simulink model "CommanderBlock"  (R2020b)
settings: Solver=VariableStepAuto  StartTime=0.0  StopTime=10.0  RelTol=1e-3
undefined symbols (not defined in the file or in its folder): cam_control_gain, l_stick_x_gain, l_stick_y_gain, m, r_stick_x_gain, r_stick_y_gain, x_final, y_final, z_final
libraries: pid_lib x4, aerolibguid x1
settings Model: Creator=macra  LastModifiedBy=macra

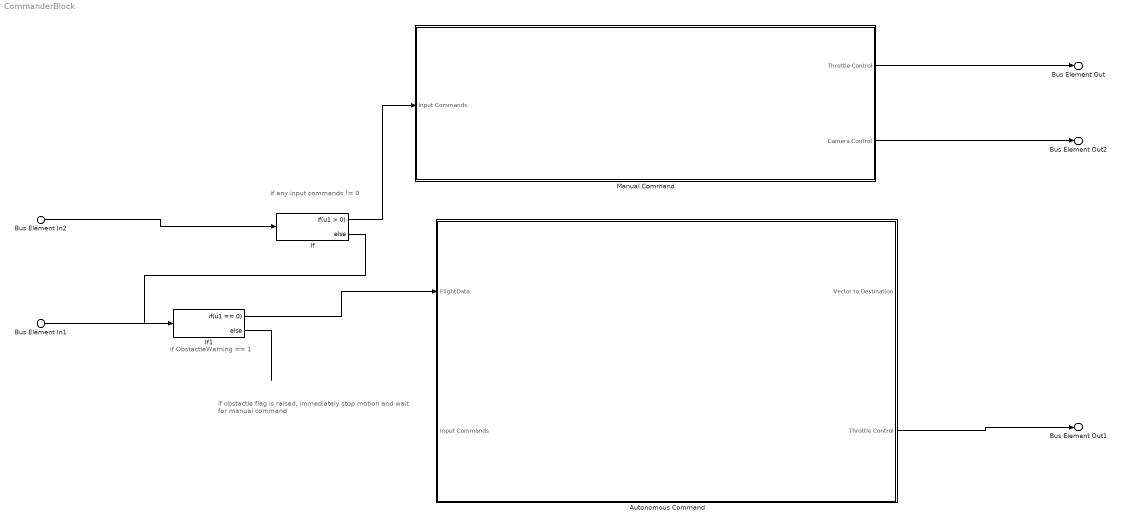
== system CommanderBlock ==
  note: if ObstactleWarning == 1
  note: if any input commands != 0
  note: if obstactle flag is raised,
      | immediately stop motion and wait for manual command
  Bus Element In2 : Inport  PortName=Input Commands
  Bus Element In1 : Inport  Port=2  PortName=Flight Data
  Autonomous Command : Subsystem
  If : If
  If1 : If  IfExpression=u1 == 0
  Manual Command : Subsystem
  Bus Element Out : Outport  PortName=Throttle Control  Element=signal1
  Bus Element Out1 : Outport  PortName=Throttle Control  Element=signal2
  Bus Element Out2 : Outport  Port=2  PortName=Camera Control  Element=signal1
  wires:
  Bus Element In2/1 -> If/1
  If/1 -> Manual Command/1(Input Commands)
  If1/1 -> Autonomous Command/1(FlightData)
  If1/2 -> ?
  Bus Element In1/1 -> If1/1
  Manual Command/1(Throttle Control) -> Bus Element Out/1
  Autonomous Command/2(Throttle Control) -> Bus Element Out1/1
  Manual Command/2(Camera Control) -> Bus Element Out2/1
  If/2 -> ?

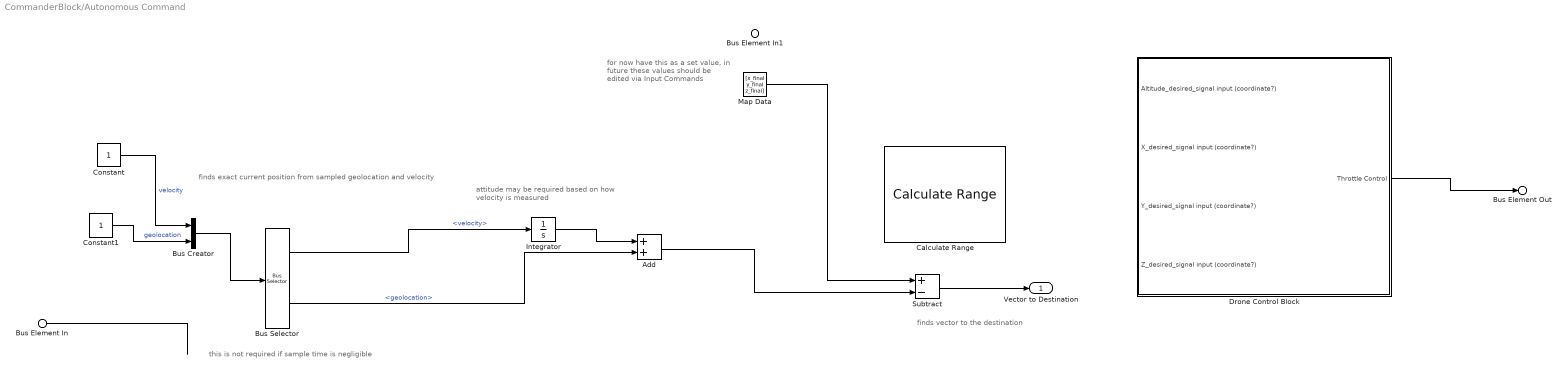
== system CommanderBlock/Autonomous Command ==
  note: finds vector to the destination
  note: finds exact current position from sampled geolocation and velocity
  note: this is not required if sample time is negligible
  note: attitude may be required based on how
      | velocity is measured
  note: for now have this as a set value,
      | in future these values should be
      | edited via Input Commands
  Bus Element In : Inport  PortName=FlightData
  Bus Element In1 : Inport  Port=2  PortName=Input Commands
  Add : Sum
  Bus Creator : BusCreator  Inputs=2
  Bus Selector : BusSelector  OutputSignals=velocity,geolocation
  Calculate Range : aerolibguid/Calculate Range
      settings: SourceProductBaseCode=AE
  Constant : Constant
  Constant1 : Constant
  Drone Control Block : Subsystem
  Integrator : Integrator
  Map Data : Constant  Value=[x_final y_final z_final]
  Subtract : Sum  Inputs=+-
  Vector to Destination : Outport
  Bus Element Out : Outport  Port=2  PortName=Throttle Control  Element=signal1
  wires:
  Constant/1 -> Bus Creator/1  "velocity"
  Bus Creator/1 -> Bus Selector/1
  Bus Selector/1 -> Integrator/1  "<velocity>"
  Constant1/1 -> Bus Creator/2  "geolocation"
  Bus Selector/2 -> Add/2  "<geolocation>"
  Integrator/1 -> Add/1
  Bus Element In/1 -> ?
  Subtract/1 -> Vector to Destination/1
  Add/1 -> Subtract/2
  Drone Control Block/1(Throttle Control) -> Bus Element Out/1
  Map Data/1 -> Subtract/1

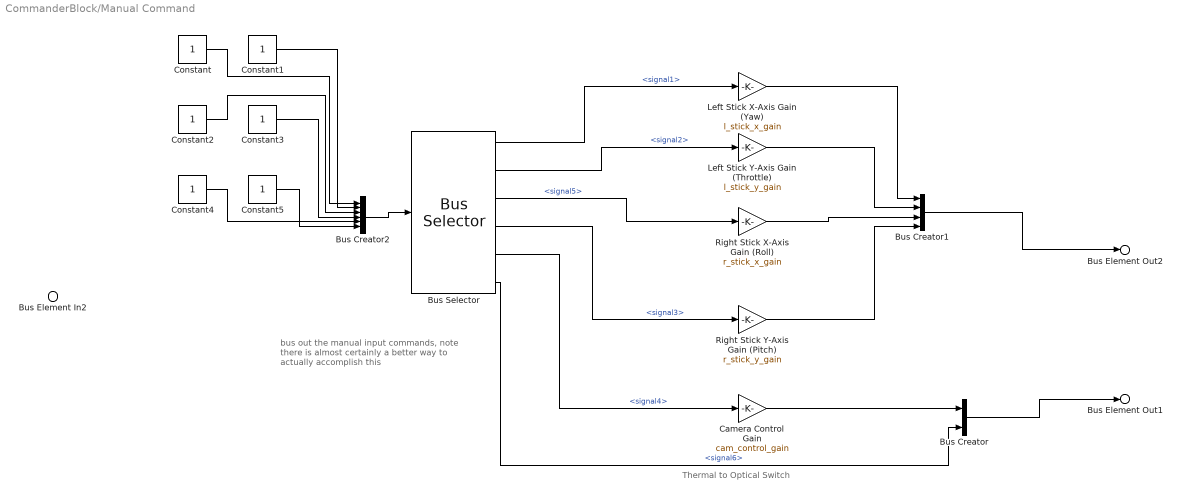
== system CommanderBlock/Manual Command ==
  note: Thermal to Optical Switch
  note: bus out the manual input commands,
      | note there is almost certainly a better way
      | to actually accomplish this
  Bus Element In2 : Inport  PortName=Input Commands
  Bus Creator : BusCreator  Inputs=2
  Bus Creator1 : BusCreator  Inputs=4
  Bus Creator2 : BusCreator  Inputs=6
  Bus Selector : BusSelector  OutputSignals=signal1,signal2,signal5,signal3,signal4,signal6
  Camera Control Gain : Gain  Gain=cam_control_gain
  Constant{,1..5} (6 alike) : Constant
  Left Stick X-Axis Gain (Yaw) : Gain  Gain=l_stick_x_gain
  Left Stick Y-Axis Gain (Throttle) : Gain  Gain=l_stick_y_gain
  Right Stick X-Axis Gain (Roll) : Gain  Gain=r_stick_x_gain
  Right Stick Y-Axis Gain (Pitch) : Gain  Gain=r_stick_y_gain
  Bus Element Out2 : Outport  PortName=Throttle Control
  Bus Element Out1 : Outport  Port=2  PortName=Camera Control
  wires:
  Constant4/1 -> Bus Creator2/5
  Constant5/1 -> Bus Creator2/6
  Bus Creator1/1 -> Bus Element Out2/1
  Bus Selector/6 -> Bus Creator/2  "<signal6>"
  Constant/1 -> Bus Creator2/1
  Constant3/1 -> Bus Creator2/4
  Right Stick Y-Axis Gain (Pitch)/1 -> Bus Creator1/4
  Bus Selector/3 -> Right Stick X-Axis Gain (Roll)/1  "<signal5>"
  Left Stick Y-Axis Gain (Throttle)/1 -> Bus Creator1/2
  Bus Selector/4 -> Right Stick Y-Axis Gain (Pitch)/1  "<signal3>"
  Bus Selector/1 -> Left Stick X-Axis Gain (Yaw)/1  "<signal1>"
  Constant1/1 -> Bus Creator2/2
  Bus Creator2/1 -> Bus Selector/1
  Bus Selector/5 -> Camera Control Gain/1  "<signal4>"
  Bus Creator/1 -> Bus Element Out1/1
  Left Stick X-Axis Gain (Yaw)/1 -> Bus Creator1/1
  Right Stick X-Axis Gain (Roll)/1 -> Bus Creator1/3
  Constant2/1 -> Bus Creator2/3
  Bus Selector/2 -> Left Stick Y-Axis Gain (Throttle)/1  "<signal2>"
  Camera Control Gain/1 -> Bus Creator/1

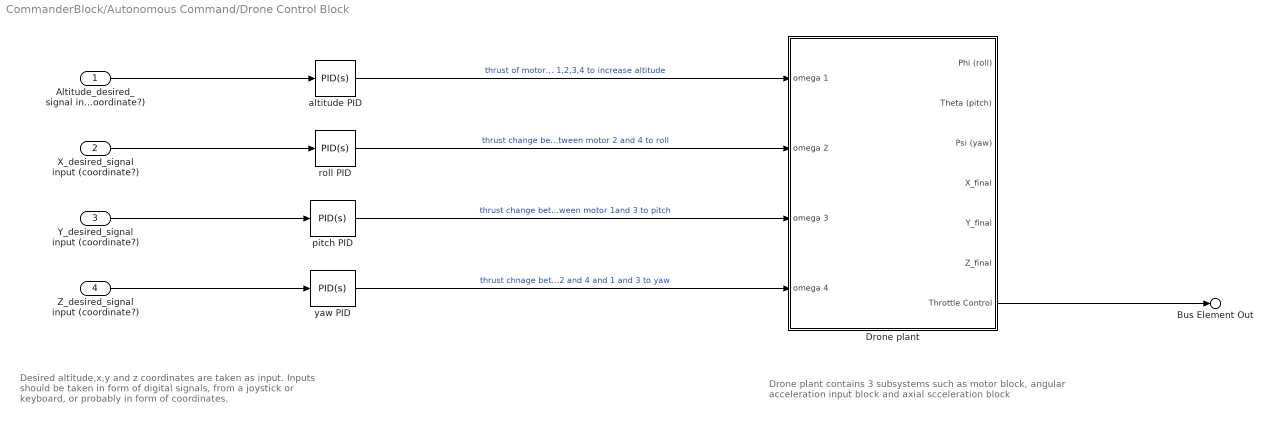
== system CommanderBlock/Autonomous Command/Drone Control Block ==
  note: Desired altitude,x,y and z coordinates are taken as input.
      | Inputs should be taken in form of digital signals,
      | from a joystick or keyboard, or probably in form of coordinates.
  note: Drone plant contains 3 subsystems such as motor block,
      | angular acceleration input block and axial scceleration block
  Altitude_desired_signal input (coordinate?) : Inport
  X_desired_signal input (coordinate?) : Inport  Port=2
  Y_desired_signal input (coordinate?) : Inport  Port=3
  Z_desired_signal input (coordinate?) : Inport  Port=4
  Drone plant : Subsystem
  altitude PID : pid_lib/PID Controller  Controller=PID  Form=Parallel  TimeDomain=Continuous-time  UseExternalTs=off  SampleTime=-1  IntegratorMethod=Forward Euler  FilterMethod=Forward Euler  ControllerParametersSource=internal  P=1  I=1  D=0  UseFilter=on  N=100  TunerSelectOption=Transfer Function Based (PID Tuner App)  InitialConditionSource=internal  InitialConditionForIntegrator=0  InitialConditionForFilter=0  DifferentiatorICPrevScaledInput=0  ExternalReset=none  TrackingMode=off  Kt=1  LimitOutput=off  SatLimitsSource=internal  UpperSaturationLimit=inf  LowerSaturationLimit=-inf  LinearizeAsGain=on  AntiWindupMode=none  Kb=1  POutMin=[]  POutMax=[]  IOutMin=[]  IOutMax=[]  DOutMin=[]  DOutMax=[]  NOutMin=[]  NOutMax=[]  SumOutMin=[]  SumOutMax=[]  SaturationOutMin=[]  SaturationOutMax=[]  PParamMin=[]  PParamMax=[]  IParamMin=[]  IParamMax=[]  DParamMin=[]  DParamMax=[]  NParamMin=[]  NParamMax=[]  KbParamMin=[]  KbParamMax=[]  KtParamMin=[]  KtParamMax=[]  KbOutMin=[]  KbOutMax=[]  KtOutMin=[]  KtOutMax=[]  IntegratorOutMin=[]  IntegratorOutMax=[]  FilterOutMin=[]  FilterOutMax=[]  SumI1OutMin=[]  SumI1OutMax=[]  SumI2OutMin=[]  SumI2OutMax=[]  SumI3OutMin=[]  SumI3OutMax=[]  SumI4OutMin=[]  SumI4OutMax=[]  SumDOutMin=[]  SumDOutMax=[]  DifferentiatorOutMin=[]  DifferentiatorOutMax=[]  FilterDiffOutCoefMin=[]  FilterDiffOutCoefMax=[]  ReciprocalOutMin=[]  ReciprocalOutMax=[]  SumDenOutMin=[]  SumDenOutMax=[]  SumNumOutMin=[]  SumNumOutMax=[]  DivideOutMin=[]  DivideOutMax=[]  UdiffTsProdOutMin=[]  UdiffTsProdOutMax=[]  NTsProdOutMin=[]  NTsProdOutMax=[]  UintegralTsProdOutMin=[]  UintegralTsProdOutMax=[]  UngainTsProdOutMin=[]  UngainTsProdOutMax=[]  IntegratorContinuousStateAttributes=''  IntegratorStateMustResolveToSignalObject=off  IntegratorRTWStateStorageClass=Auto  FilterContinuousStateAttributes=''  FilterStateMustResolveToSignalObject=off  FilterRTWStateStorageClass=Auto  ParallelPVariant=InternalParameters  IdealPVariant=Disabled  IVariant=InternalParameters  DVariant=InternalParameters  IntegratorVariant=Continuous  SatVariant=Disabled  AWVariant=Passthrough  PCopyVariant=Disabled  TRVariant=Disabled  FdbkBlocksVariant=Forward  IdealPFdbkVariant=Disabled  SatFdbkVariant=Disabled  DerivativeFilterVariant=ContFilter  NVariant=InternalParameters  NCopyVariant=Disabled  FilterICVariant=InternalICsFilter  IntegratorICVariant=InternalICs  ExternalResetVariant=Disabled  TRSumVariant=Passthrough  SumFdbkVariant=Disabled  SumVariant=Sum_PID  TsampFilterVariant=InternalTs  TsampNgainVariant=Passthrough  TsampIntegralVariant=Passthrough  ExternalSaturationOutDataTypeStr=Inherit: Same as second input
  pitch PID : pid_lib/PID Controller  Controller=PID  Form=Parallel  TimeDomain=Continuous-time  UseExternalTs=off  SampleTime=-1  IntegratorMethod=Forward Euler  FilterMethod=Forward Euler  ControllerParametersSource=internal  P=1  I=1  D=0  UseFilter=on  N=100  TunerSelectOption=Transfer Function Based (PID Tuner App)  InitialConditionSource=internal  InitialConditionForIntegrator=0  InitialConditionForFilter=0  DifferentiatorICPrevScaledInput=0  ExternalReset=none  TrackingMode=off  Kt=1  LimitOutput=off  SatLimitsSource=internal  UpperSaturationLimit=inf  LowerSaturationLimit=-inf  LinearizeAsGain=on  AntiWindupMode=none  Kb=1  POutMin=[]  POutMax=[]  IOutMin=[]  IOutMax=[]  DOutMin=[]  DOutMax=[]  NOutMin=[]  NOutMax=[]  SumOutMin=[]  SumOutMax=[]  SaturationOutMin=[]  SaturationOutMax=[]  PParamMin=[]  PParamMax=[]  IParamMin=[]  IParamMax=[]  DParamMin=[]  DParamMax=[]  NParamMin=[]  NParamMax=[]  KbParamMin=[]  KbParamMax=[]  KtParamMin=[]  KtParamMax=[]  KbOutMin=[]  KbOutMax=[]  KtOutMin=[]  KtOutMax=[]  IntegratorOutMin=[]  IntegratorOutMax=[]  FilterOutMin=[]  FilterOutMax=[]  SumI1OutMin=[]  SumI1OutMax=[]  SumI2OutMin=[]  SumI2OutMax=[]  SumI3OutMin=[]  SumI3OutMax=[]  SumI4OutMin=[]  SumI4OutMax=[]  SumDOutMin=[]  SumDOutMax=[]  DifferentiatorOutMin=[]  DifferentiatorOutMax=[]  FilterDiffOutCoefMin=[]  FilterDiffOutCoefMax=[]  ReciprocalOutMin=[]  ReciprocalOutMax=[]  SumDenOutMin=[]  SumDenOutMax=[]  SumNumOutMin=[]  SumNumOutMax=[]  DivideOutMin=[]  DivideOutMax=[]  UdiffTsProdOutMin=[]  UdiffTsProdOutMax=[]  NTsProdOutMin=[]  NTsProdOutMax=[]  UintegralTsProdOutMin=[]  UintegralTsProdOutMax=[]  UngainTsProdOutMin=[]  UngainTsProdOutMax=[]  IntegratorContinuousStateAttributes=''  IntegratorStateMustResolveToSignalObject=off  IntegratorRTWStateStorageClass=Auto  FilterContinuousStateAttributes=''  FilterStateMustResolveToSignalObject=off  FilterRTWStateStorageClass=Auto  ParallelPVariant=InternalParameters  IdealPVariant=Disabled  IVariant=InternalParameters  DVariant=InternalParameters  IntegratorVariant=Continuous  SatVariant=Disabled  AWVariant=Passthrough  PCopyVariant=Disabled  TRVariant=Disabled  FdbkBlocksVariant=Forward  IdealPFdbkVariant=Disabled  SatFdbkVariant=Disabled  DerivativeFilterVariant=ContFilter  NVariant=InternalParameters  NCopyVariant=Disabled  FilterICVariant=InternalICsFilter  IntegratorICVariant=InternalICs  ExternalResetVariant=Disabled  TRSumVariant=Passthrough  SumFdbkVariant=Disabled  SumVariant=Sum_PID  TsampFilterVariant=InternalTs  TsampNgainVariant=Passthrough  TsampIntegralVariant=Passthrough  ExternalSaturationOutDataTypeStr=Inherit: Same as second input
  roll PID : pid_lib/PID Controller  Controller=PID  Form=Parallel  TimeDomain=Continuous-time  UseExternalTs=off  SampleTime=-1  IntegratorMethod=Forward Euler  FilterMethod=Forward Euler  ControllerParametersSource=internal  P=1  I=1  D=0  UseFilter=on  N=100  TunerSelectOption=Transfer Function Based (PID Tuner App)  InitialConditionSource=internal  InitialConditionForIntegrator=0  InitialConditionForFilter=0  DifferentiatorICPrevScaledInput=0  ExternalReset=none  TrackingMode=off  Kt=1  LimitOutput=off  SatLimitsSource=internal  UpperSaturationLimit=inf  LowerSaturationLimit=-inf  LinearizeAsGain=on  AntiWindupMode=none  Kb=1  POutMin=[]  POutMax=[]  IOutMin=[]  IOutMax=[]  DOutMin=[]  DOutMax=[]  NOutMin=[]  NOutMax=[]  SumOutMin=[]  SumOutMax=[]  SaturationOutMin=[]  SaturationOutMax=[]  PParamMin=[]  PParamMax=[]  IParamMin=[]  IParamMax=[]  DParamMin=[]  DParamMax=[]  NParamMin=[]  NParamMax=[]  KbParamMin=[]  KbParamMax=[]  KtParamMin=[]  KtParamMax=[]  KbOutMin=[]  KbOutMax=[]  KtOutMin=[]  KtOutMax=[]  IntegratorOutMin=[]  IntegratorOutMax=[]  FilterOutMin=[]  FilterOutMax=[]  SumI1OutMin=[]  SumI1OutMax=[]  SumI2OutMin=[]  SumI2OutMax=[]  SumI3OutMin=[]  SumI3OutMax=[]  SumI4OutMin=[]  SumI4OutMax=[]  SumDOutMin=[]  SumDOutMax=[]  DifferentiatorOutMin=[]  DifferentiatorOutMax=[]  FilterDiffOutCoefMin=[]  FilterDiffOutCoefMax=[]  ReciprocalOutMin=[]  ReciprocalOutMax=[]  SumDenOutMin=[]  SumDenOutMax=[]  SumNumOutMin=[]  SumNumOutMax=[]  DivideOutMin=[]  DivideOutMax=[]  UdiffTsProdOutMin=[]  UdiffTsProdOutMax=[]  NTsProdOutMin=[]  NTsProdOutMax=[]  UintegralTsProdOutMin=[]  UintegralTsProdOutMax=[]  UngainTsProdOutMin=[]  UngainTsProdOutMax=[]  IntegratorContinuousStateAttributes=''  IntegratorStateMustResolveToSignalObject=off  IntegratorRTWStateStorageClass=Auto  FilterContinuousStateAttributes=''  FilterStateMustResolveToSignalObject=off  FilterRTWStateStorageClass=Auto  ParallelPVariant=InternalParameters  IdealPVariant=Disabled  IVariant=InternalParameters  DVariant=InternalParameters  IntegratorVariant=Continuous  SatVariant=Disabled  AWVariant=Passthrough  PCopyVariant=Disabled  TRVariant=Disabled  FdbkBlocksVariant=Forward  IdealPFdbkVariant=Disabled  SatFdbkVariant=Disabled  DerivativeFilterVariant=ContFilter  NVariant=InternalParameters  NCopyVariant=Disabled  FilterICVariant=InternalICsFilter  IntegratorICVariant=InternalICs  ExternalResetVariant=Disabled  TRSumVariant=Passthrough  SumFdbkVariant=Disabled  SumVariant=Sum_PID  TsampFilterVariant=InternalTs  TsampNgainVariant=Passthrough  TsampIntegralVariant=Passthrough  ExternalSaturationOutDataTypeStr=Inherit: Same as second input
  yaw PID : pid_lib/PID Controller  Controller=PID  Form=Parallel  TimeDomain=Continuous-time  UseExternalTs=off  SampleTime=-1  IntegratorMethod=Forward Euler  FilterMethod=Forward Euler  ControllerParametersSource=internal  P=1  I=1  D=0  UseFilter=on  N=100  TunerSelectOption=Transfer Function Based (PID Tuner App)  InitialConditionSource=internal  InitialConditionForIntegrator=0  InitialConditionForFilter=0  DifferentiatorICPrevScaledInput=0  ExternalReset=none  TrackingMode=off  Kt=1  LimitOutput=off  SatLimitsSource=internal  UpperSaturationLimit=inf  LowerSaturationLimit=-inf  LinearizeAsGain=on  AntiWindupMode=none  Kb=1  POutMin=[]  POutMax=[]  IOutMin=[]  IOutMax=[]  DOutMin=[]  DOutMax=[]  NOutMin=[]  NOutMax=[]  SumOutMin=[]  SumOutMax=[]  SaturationOutMin=[]  SaturationOutMax=[]  PParamMin=[]  PParamMax=[]  IParamMin=[]  IParamMax=[]  DParamMin=[]  DParamMax=[]  NParamMin=[]  NParamMax=[]  KbParamMin=[]  KbParamMax=[]  KtParamMin=[]  KtParamMax=[]  KbOutMin=[]  KbOutMax=[]  KtOutMin=[]  KtOutMax=[]  IntegratorOutMin=[]  IntegratorOutMax=[]  FilterOutMin=[]  FilterOutMax=[]  SumI1OutMin=[]  SumI1OutMax=[]  SumI2OutMin=[]  SumI2OutMax=[]  SumI3OutMin=[]  SumI3OutMax=[]  SumI4OutMin=[]  SumI4OutMax=[]  SumDOutMin=[]  SumDOutMax=[]  DifferentiatorOutMin=[]  DifferentiatorOutMax=[]  FilterDiffOutCoefMin=[]  FilterDiffOutCoefMax=[]  ReciprocalOutMin=[]  ReciprocalOutMax=[]  SumDenOutMin=[]  SumDenOutMax=[]  SumNumOutMin=[]  SumNumOutMax=[]  DivideOutMin=[]  DivideOutMax=[]  UdiffTsProdOutMin=[]  UdiffTsProdOutMax=[]  NTsProdOutMin=[]  NTsProdOutMax=[]  UintegralTsProdOutMin=[]  UintegralTsProdOutMax=[]  UngainTsProdOutMin=[]  UngainTsProdOutMax=[]  IntegratorContinuousStateAttributes=''  IntegratorStateMustResolveToSignalObject=off  IntegratorRTWStateStorageClass=Auto  FilterContinuousStateAttributes=''  FilterStateMustResolveToSignalObject=off  FilterRTWStateStorageClass=Auto  ParallelPVariant=InternalParameters  IdealPVariant=Disabled  IVariant=InternalParameters  DVariant=InternalParameters  IntegratorVariant=Continuous  SatVariant=Disabled  AWVariant=Passthrough  PCopyVariant=Disabled  TRVariant=Disabled  FdbkBlocksVariant=Forward  IdealPFdbkVariant=Disabled  SatFdbkVariant=Disabled  DerivativeFilterVariant=ContFilter  NVariant=InternalParameters  NCopyVariant=Disabled  FilterICVariant=InternalICsFilter  IntegratorICVariant=InternalICs  ExternalResetVariant=Disabled  TRSumVariant=Passthrough  SumFdbkVariant=Disabled  SumVariant=Sum_PID  TsampFilterVariant=InternalTs  TsampNgainVariant=Passthrough  TsampIntegralVariant=Passthrough  ExternalSaturationOutDataTypeStr=Inherit: Same as second input
  Bus Element Out : Outport  PortName=Throttle Control  Element=signal1
  wires:
  Altitude_desired_signal input (coordinate?)/1 -> altitude PID/1
  pitch PID/1 -> Drone plant/3(omega 3)  "thrust change between motor 1and 3 to pitch"
  Y_desired_signal input (coordinate?)/1 -> pitch PID/1
  yaw PID/1 -> Drone plant/4(omega 4)  "thrust chnage between motor 2 and 4 and 1 and 3 to yaw"
  Drone plant/7(Throttle Control) -> Bus Element Out/1
  Z_desired_signal input (coordinate?)/1 -> yaw PID/1
  X_desired_signal input (coordinate?)/1 -> roll PID/1
  roll PID/1 -> Drone plant/2(omega 2)  "thrust change between motor 2 and 4 to roll"
  altitude PID/1 -> Drone plant/1(omega 1)  "thrust of motor 1,2,3,4 to increase altitude"

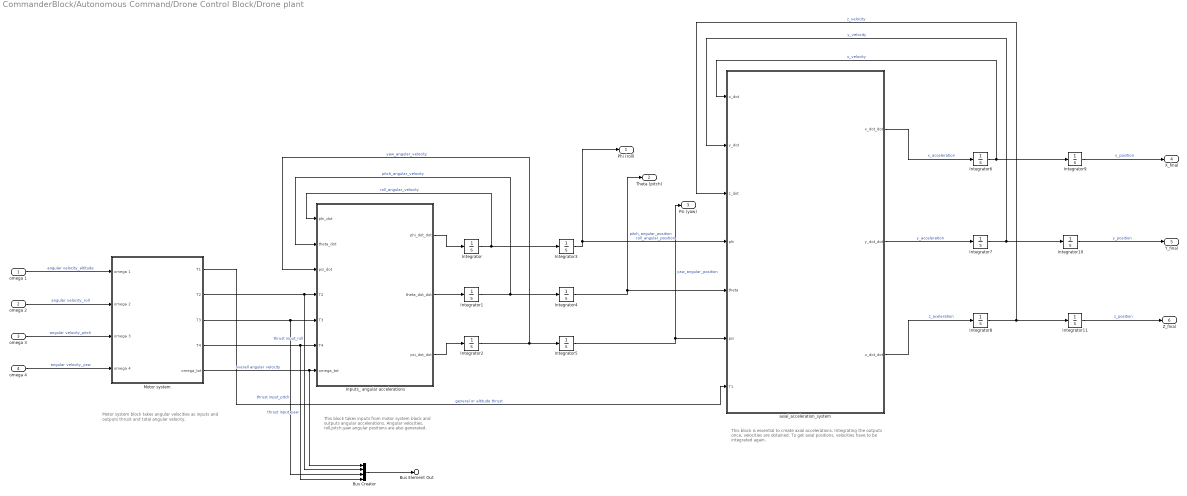
== system CommanderBlock/Autonomous Command/Drone Control Block/Drone plant ==
  note: This block is essential to create axial accelerations. Integrating the outputs
      | once, velocities are obtained. To get axial positions, velocities have to be
      | integrated again.
  note: This block takes inputs from motor system block
      | and outputs angular accelerations. Angular velocities,
      | roll,pitch,yaw angular positions are also generated.
  note: Motor system block takes angular velocities as inputs
      | and outputs thrust and total angular velocity.
  omega 1 : Inport
  omega 2 : Inport  Port=2
  omega 3 : Inport  Port=3
  omega 4 : Inport  Port=4
  Bus Creator : BusCreator  Inputs=4
  Inputs_ angular accelerations : Subsystem
  Integrator{,1..11} (12 alike) : Integrator
  Motor system : Subsystem
  axial_acceleration_system : Subsystem
  Phi (roll) : Outport
  Theta (pitch) : Outport  Port=2
  Psi (yaw) : Outport  Port=3
  X_final : Outport  Port=4
  Y_final : Outport  Port=5
  Z_final : Outport  Port=6
  Bus Element Out : Outport  Port=7  PortName=Throttle Control  Element=signal1
  wires:
  omega 1/1 -> Motor system/1(omega 1)  "angular velocity_altitude"
  omega 2/1 -> Motor system/2(omega 2)  "angular velocity_roll"
  omega 3/1 -> Motor system/3(omega 3)  "angular velocity_pitch"
  omega 4/1 -> Motor system/4(omega 4)  "angular velocity_yaw"
  Motor system/5(omega_tot) -> Bus Creator/1, Inputs_ angular accelerations/7(omega_tot)  "overall angular velocity"
  Motor system/2(T2) -> Bus Creator/2, Inputs_ angular accelerations/4(T2)  "thrust input_roll"
  Motor system/3(T3) -> Bus Creator/3, Inputs_ angular accelerations/5(T3)  "thrust input_pitch"
  Motor system/4(T4) -> Bus Creator/4, Inputs_ angular accelerations/6(T4)  "thrust input_yaw"
  Motor system/1(T1) -> axial_acceleration_system/7(T1)  "general or altitude thrust"
  Inputs_ angular accelerations/1(phi_dot_dot) -> Integrator/1
  Integrator/1 -> Inputs_ angular accelerations/1(phi_dot), Integrator3/1  "roll_angular_velocity"
  Integrator1/1 -> Inputs_ angular accelerations/2(theta_dot), Integrator4/1  "pitch_angular_velocity"
  Integrator2/1 -> Inputs_ angular accelerations/3(psi_dot), Integrator5/1  "yaw_angular_velocity"
  Inputs_ angular accelerations/2(theta_dot_dot) -> Integrator1/1
  Inputs_ angular accelerations/3(psi_dot_dot) -> Integrator2/1
  Integrator4/1 -> Theta (pitch)/1, axial_acceleration_system/5(theta)  "pitch_angular_position"
  Integrator3/1 -> Phi (roll)/1, axial_acceleration_system/4(phi)  "roll_angular_position"
  Integrator5/1 -> axial_acceleration_system/6(psi), Psi (yaw)/1  "yaw_angular_position"
  axial_acceleration_system/1(x_dot_dot) -> Integrator6/1  "x_acceleration"
  axial_acceleration_system/2(y_dot_dot) -> Integrator7/1  "y_acceleration"
  axial_acceleration_system/3(z_dot_dot) -> Integrator8/1  "z_aceleration"
  Integrator6/1 -> axial_acceleration_system/1(x_dot), Integrator9/1  "x_velocity"
  Integrator9/1 -> X_final/1  "x_position"
  Integrator7/1 -> axial_acceleration_system/2(y_dot), Integrator10/1  "y_velocity"
  Integrator10/1 -> Y_final/1  "y_position"
  Integrator8/1 -> axial_acceleration_system/3(z_dot), Integrator11/1  "z_velocity"
  Integrator11/1 -> Z_final/1  "z_position"
  Bus Creator/1 -> Bus Element Out/1

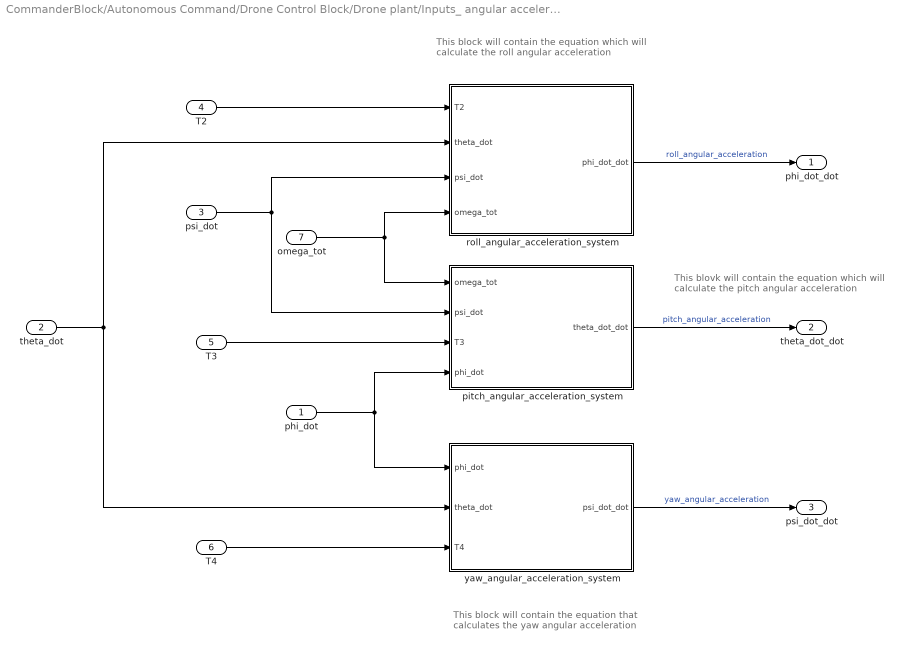
== system CommanderBlock/Autonomous Command/Drone Control Block/Drone plant/Inputs_ angular accelerations ==
  note: This blovk will contain the equation
      | which will calculate the pitch angular acceleration
  note: This block will contain the equation
      | that calculates the yaw angular acceleration
  note: This block will contain the equation
      | which will calculate the roll angular acceleration
  phi_dot : Inport
  theta_dot : Inport  Port=2
  psi_dot : Inport  Port=3
  T2 : Inport  Port=4
  T3 : Inport  Port=5
  T4 : Inport  Port=6
  omega_tot : Inport  Port=7
  pitch_angular_acceleration_system : Subsystem
  roll_angular_acceleration_system : Subsystem
  yaw_angular_acceleration_system : Subsystem
  phi_dot_dot : Outport
  theta_dot_dot : Outport  Port=2
  psi_dot_dot : Outport  Port=3
  wires:
  roll_angular_acceleration_system/1(phi_dot_dot) -> phi_dot_dot/1  "roll_angular_acceleration"
  pitch_angular_acceleration_system/1(theta_dot_dot) -> theta_dot_dot/1  "pitch_angular_acceleration"
  yaw_angular_acceleration_system/1(psi_dot_dot) -> psi_dot_dot/1  "yaw_angular_acceleration"
  T2/1 -> roll_angular_acceleration_system/1(T2)
  theta_dot/1 -> yaw_angular_acceleration_system/2(theta_dot), roll_angular_acceleration_system/2(theta_dot)
  psi_dot/1 -> roll_angular_acceleration_system/3(psi_dot), pitch_angular_acceleration_system/2(psi_dot)
  T3/1 -> pitch_angular_acceleration_system/3(T3)
  T4/1 -> yaw_angular_acceleration_system/3(T4)
  phi_dot/1 -> yaw_angular_acceleration_system/1(phi_dot), pitch_angular_acceleration_system/4(phi_dot)
  omega_tot/1 -> pitch_angular_acceleration_system/1(omega_tot), roll_angular_acceleration_system/4(omega_tot)

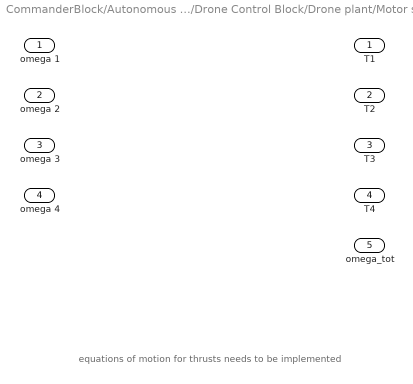
== system CommanderBlock/Autonomous Command/Drone Control Block/Drone plant/Motor system ==
  note: equations of motion for thrusts needs to be implemented
  omega 1 : Inport
  omega 2 : Inport  Port=2
  omega 3 : Inport  Port=3
  omega 4 : Inport  Port=4
  T1 : Outport
  T2 : Outport  Port=2
  T3 : Outport  Port=3
  T4 : Outport  Port=4
  omega_tot : Outport  Port=5

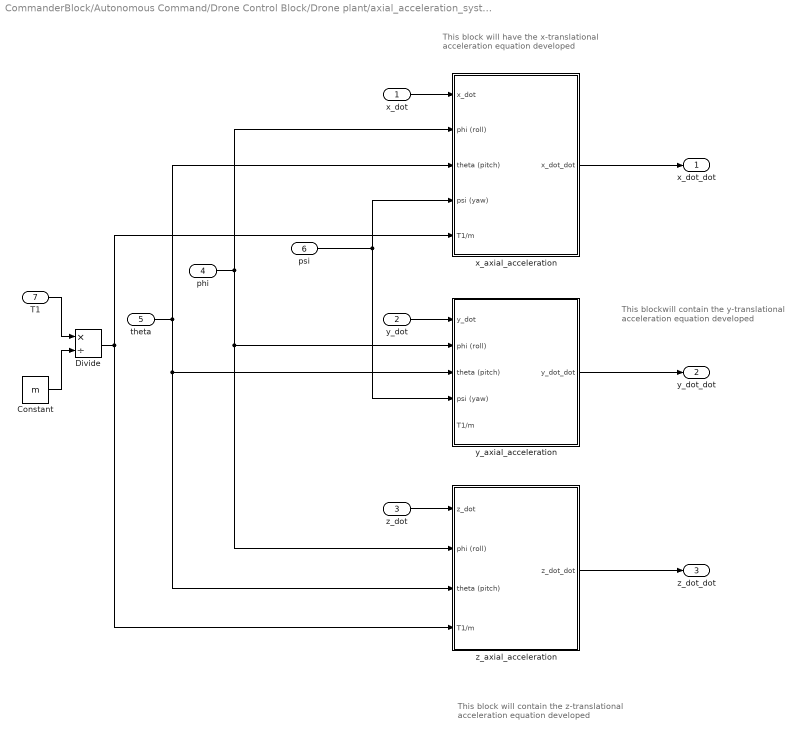
== system CommanderBlock/Autonomous Command/Drone Control Block/Drone plant/axial_acceleration_system ==
  note: This block will contain the z-translational
      | acceleration equation developed
  note: This blockwill contain the y-translational
      | acceleration equation developed
  note: This block will have the x-translational
      | acceleration equation developed
  x_dot : Inport
  y_dot : Inport  Port=2
  z_dot : Inport  Port=3
  phi : Inport  Port=4
  theta : Inport  Port=5
  psi : Inport  Port=6
  T1 : Inport  Port=7
  Constant : Constant  Value=m
  Divide : Product  Inputs=*/
  x_axial_acceleration : Subsystem
  y_axial_acceleration : Subsystem
  z_axial_acceleration : Subsystem
  x_dot_dot : Outport
  y_dot_dot : Outport  Port=2
  z_dot_dot : Outport  Port=3
  wires:
  x_axial_acceleration/1(x_dot_dot) -> x_dot_dot/1
  z_axial_acceleration/1(z_dot_dot) -> z_dot_dot/1
  y_axial_acceleration/1(y_dot_dot) -> y_dot_dot/1
  x_dot/1 -> x_axial_acceleration/1(x_dot)
  y_dot/1 -> y_axial_acceleration/1(y_dot)
  z_dot/1 -> z_axial_acceleration/1(z_dot)
  phi/1 -> y_axial_acceleration/2(phi (roll)), z_axial_acceleration/2(phi (roll)), x_axial_acceleration/2(phi (roll))
  theta/1 -> x_axial_acceleration/3(theta (pitch)), y_axial_acceleration/3(theta (pitch)), z_axial_acceleration/3(theta (pitch))
  psi/1 -> x_axial_acceleration/4(psi (yaw)), y_axial_acceleration/4(psi (yaw))
  Constant/1 -> Divide/2
  T1/1 -> Divide/1
  Divide/1 -> z_axial_acceleration/4(T1/m), x_axial_acceleration/5(T1/m)

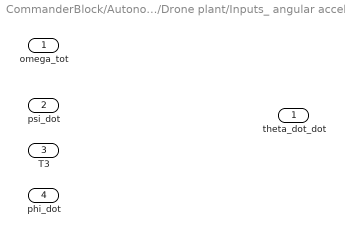
== system CommanderBlock/Autonomous Command/Drone Control Block/Drone plant/Inputs_ angular accelerations/pitch_angular_acceleration_system ==
  omega_tot : Inport
  psi_dot : Inport  Port=2
  T3 : Inport  Port=3
  phi_dot : Inport  Port=4
  theta_dot_dot : Outport

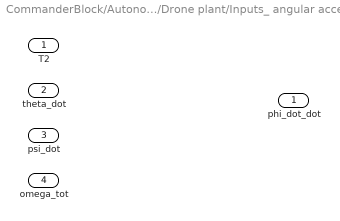
== system CommanderBlock/Autonomous Command/Drone Control Block/Drone plant/Inputs_ angular accelerations/roll_angular_acceleration_system ==
  T2 : Inport
  theta_dot : Inport  Port=2
  psi_dot : Inport  Port=3
  omega_tot : Inport  Port=4
  phi_dot_dot : Outport

== system CommanderBlock/Autonomous Command/Drone Control Block/Drone plant/Inputs_ angular accelerations/yaw_angular_acceleration_system ==
  phi_dot : Inport
  theta_dot : Inport  Port=2
  T4 : Inport  Port=3
  psi_dot_dot : Outport

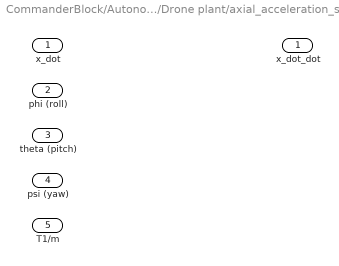
== system CommanderBlock/Autonomous Command/Drone Control Block/Drone plant/axial_acceleration_system/x_axial_acceleration ==
  x_dot : Inport
  phi (roll) : Inport  Port=2
  theta (pitch) : Inport  Port=3
  psi (yaw) : Inport  Port=4
  T1/m : Inport  Port=5
  x_dot_dot : Outport

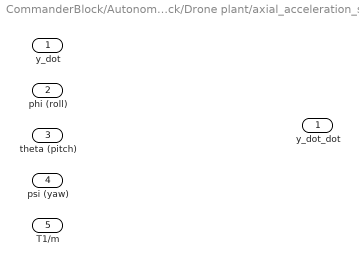
== system CommanderBlock/Autonomous Command/Drone Control Block/Drone plant/axial_acceleration_system/y_axial_acceleration ==
  y_dot : Inport
  phi (roll) : Inport  Port=2
  theta (pitch) : Inport  Port=3
  psi (yaw) : Inport  Port=4
  T1/m : Inport  Port=5
  y_dot_dot : Outport

== system CommanderBlock/Autonomous Command/Drone Control Block/Drone plant/axial_acceleration_system/z_axial_acceleration ==
  z_dot : Inport
  phi (roll) : Inport  Port=2
  theta (pitch) : Inport  Port=3
  T1/m : Inport  Port=4
  z_dot_dot : Outport
